simulink model "elec3200hw5"  (R2016a)
settings: Solver=VariableStepAuto  StartTime=0.0  StopTime=10.0  RelTol=1e-3
settings Model: Creator=古乔  LastModifiedBy=古乔

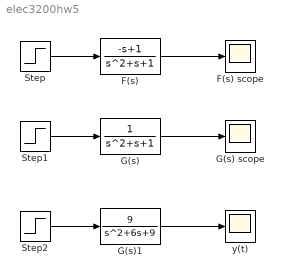
== system elec3200hw5 ==
  F(s) : TransferFcn  Numerator=[-1 1]  Denominator=[1 1 1]
  F(s) scope : Scope
  G(s) : TransferFcn  Denominator=[1 1 1]
  G(s) scope : Scope
  G(s)1 : TransferFcn  Numerator=[9]  Denominator=[1 6 9]
  Step : Step  SampleTime=0
  Step1 : Step  SampleTime=0
  Step2 : Step  SampleTime=0
  y(t) : Scope
  wires:
  F(s)/1 -> F(s) scope/1
  Step/1 -> F(s)/1
  G(s)/1 -> G(s) scope/1
  Step1/1 -> G(s)/1
  G(s)1/1 -> y(t)/1
  Step2/1 -> G(s)1/1
